simulink model "Aula7_1"  (R2013b)
settings: Solver=ode45  StartTime=0.0  StopTime=1  RelTol=1e-3
settings Model: Creator=ThiagoCordeiro  LastModifiedBy=thiag

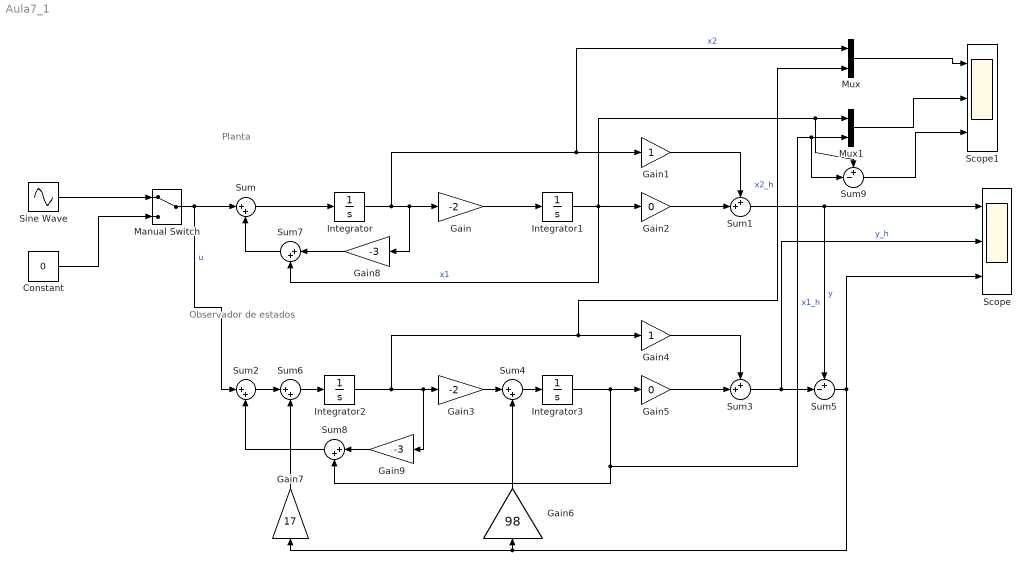
== system Aula7_1 ==
  note: Planta
  note: Observador de estados
  Constant : Constant  Value=0
  Gain : Gain  Gain=-2
  Gain1 : Gain
  Gain2 : Gain  Gain=0
  Gain3 : Gain  Gain=-2
  Gain4 : Gain
  Gain5 : Gain  Gain=0
  Gain6 : Gain  Gain=98
  Gain7 : Gain  Gain=17
  Gain8 : Gain  Gain=-3
  Gain9 : Gain  Gain=-3
  Integrator : Integrator  InitialCondition=5
  Integrator1 : Integrator  InitialCondition=1
  Integrator2 : Integrator  InitialCondition=50
  Integrator3 : Integrator  InitialCondition=10
  Manual Switch : ManualSwitch
  Mux : Mux  Inputs=2
  Mux1 : Mux  Inputs=2
  Scope : Scope  NumInputPorts=3
      settings: YMin=-5~-5~-5  YMax=5~5~5
  Scope1 : Scope  NumInputPorts=3
      settings: YMin=-5~-5~-5  YMax=5~5~5
  Sine Wave : Sin  Amplitude=10  SampleTime=0
  Sum{,2,4,6..8} (6 alike) : Sum  Inputs=|++
  Sum1 : Sum  Inputs=++|
  Sum3 : Sum  Inputs=++|
  Sum5 : Sum  Inputs=+-|
  Sum9 : Sum  Inputs=+-|
  wires:
  Sine Wave/1 -> Manual Switch/1
  Sum/1 -> Integrator/1
  Constant/1 -> Manual Switch/2
  Gain/1 -> Integrator1/1
  Integrator1/1 -> Sum9/1, Mux1/1, Gain2/1, Sum7/2  "x1"
  Gain2/1 -> Sum1/2
  Gain1/1 -> Sum1/1
  Sum1/1 -> Sum5/1, Scope/1  "y"
  Manual Switch/1 -> Sum/1, Sum2/1  "u"
  Integrator3/1 -> Sum9/2, Mux1/2, Sum8/2, Gain5/1  "x1_h"
  Gain5/1 -> Sum3/2
  Gain4/1 -> Sum3/1
  Sum3/1 -> Scope/2, Sum5/2  "y_h"
  Gain3/1 -> Sum4/1
  Sum4/1 -> Integrator3/1
  Gain6/1 -> Sum4/2
  Sum5/1 -> Scope/3, Gain6/1, Gain7/1
  Sum2/1 -> Sum6/1
  Sum6/1 -> Integrator2/1
  Gain7/1 -> Sum6/2
  Gain8/1 -> Sum7/1
  Sum7/1 -> Sum/2
  Gain9/1 -> Sum8/1
  Sum8/1 -> Sum2/2
  Integrator/1 -> Mux/1, Gain1/1, Gain8/1, Gain/1  "x2"
  Integrator2/1 -> Mux/2, Gain4/1, Gain9/1, Gain3/1  "x2_h"
  Mux/1 -> Scope1/1
  Mux1/1 -> Scope1/2
  Sum9/1 -> Scope1/3
